simulink library "Driveline_ConnectFRDiffFDiffR"  (R2019a)
settings: Solver=VariableStepAuto  StartTime=0.0  StopTime=10.0  RelTol=1e-3
undefined symbols (not defined in the file): Driveline
libraries: sm_car_lib x6, fl_lib x4, sdl_lib x2
Description:
  | Component of Simscape Vehicle Templates Library
  | 
  | Copyright 2018-2020 The MathWorks, Inc.
settings Model: Creator=smiller  LastModifiedBy=smiller
settings DataIOCC: ReturnWorkspaceOutputs=off
settings DebuggingCC: ArithmeticOperatorsInVariantConditions=warning

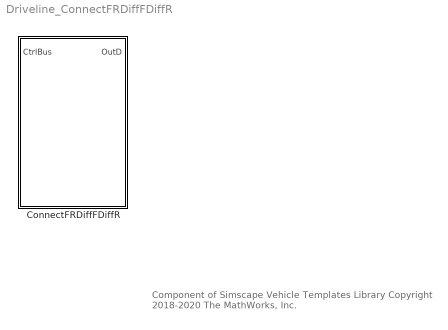
== system Driveline_ConnectFRDiffFDiffR ==
  note: Component of Simscape Vehicle Templates Library
      | Copyright 2018-2020 The MathWorks, Inc.
  ConnectFRDiffFDiffR : Subsystem  Tag=PublishSubsystem  VariantControl=ConnectFRDiffFDiffR  mask(Driveline, Connected Front and Rear){InitTriggerDropdown=0}
      mask prompts: InitTriggerDropdown "Initialization Trigger Dropdown"
      mask help: Models front and rear drivelines connected by a viscous coupling.
      mask init:
      | curblk = gcb;
      | 
      | % Trigger Mask Initialization for 
      | % variant subsystems below this level
      | sm_car_lib_maskInitTrigger(curblk);
      mask TypeOptions InitTriggerDropdown: 0 | 1
      mask Display: image('sm_car_vehicle_driveline_connectfrdifffdiffr_IMAGE.png');

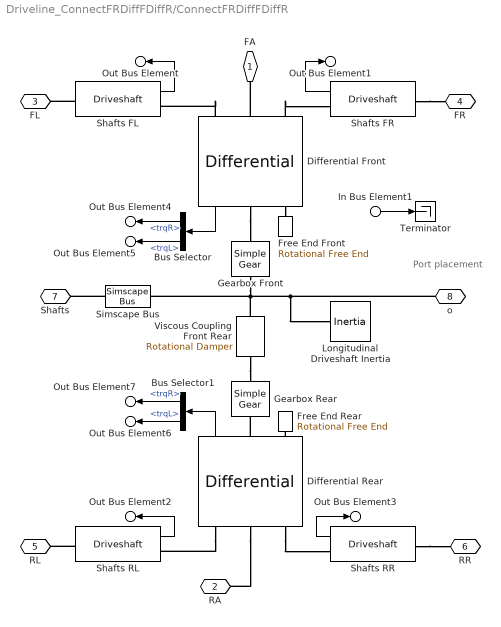
== system Driveline_ConnectFRDiffFDiffR/ConnectFRDiffFDiffR ==
  note: Port
      | placement
  In Bus Element1 : Inport  PortName=CtrlBus
  Bus Selector : BusSelector  OutputSignals=trqR,trqL
  Bus Selector1 : BusSelector  OutputSignals=trqR,trqL
  Differential Front : sm_car_lib/Driveline/Differential  VariantControl=Variant1  Differential=Driveline.DifferentialF  VariantLabel=Driveline.DifferentialF.class.Value  InitTriggerDropdown=0
      settings: AttributesFormatString=%<ActiveVariant>
  Differential Rear : sm_car_lib/Driveline/Differential  VariantControl=Variant1  Differential=Driveline.DifferentialR  VariantLabel=Driveline.DifferentialR.class.Value  InitTriggerDropdown=0
      settings: AttributesFormatString=%<ActiveVariant>
  Free End Front : fl_lib/Mechanical/Rotational Elements/Rotational Free End  w_specify=off  w_priority=None  w=0 rad/s  w_nominal_specify=off  w_nominal_unit=rad/s  w_nominal_value=1
      settings: SourceProductName=Simscape  SourceProductBaseCode=SS
  Free End Rear : fl_lib/Mechanical/Rotational Elements/Rotational Free End  w_specify=off  w_priority=None  w=0 rad/s  w_nominal_specify=off  w_nominal_unit=rad/s  w_nominal_value=1
      settings: SourceProductName=Simscape  SourceProductBaseCode=SS
  Gearbox Front : sdl_lib/Gears/Simple Gear  ratio=Driveline.GearboxF.ratio.Value  rotation_direction=1  friction_model=1  T_noload=0.1 N*m  T_nom=5 N*m  efficiency_nom=0.8  efficiency=0.8  mu_visc=[0, 0] N*m/(rad/s)  w_thr=0.01 rad/s  pwr_thr=0.001 W  enable_faults=0  efficiency_fault=0.05  external_fault=simscape.enum.onoff.off  temporal_fault=0  fault_time=5 s  fault_angles=pi / 12 rad  report_fault=1  temperature_TLU=[280, 300, 320] K  load_TLU=[1, 5, 10] N*m  efficiency_TLU=[.95, .9, .85]  efficiency_TLU2=[.85, .8, .75; .95, .9, .85; .85, .8, .7]  thermal_mass=50 J/K  T_init=300 K
      settings: SourceProductName=Simscape Driveline
  Gearbox Rear : sdl_lib/Gears/Simple Gear  ratio=Driveline.GearboxR.ratio.Value  rotation_direction=1  friction_model=1  T_noload=0.1 N*m  T_nom=5 N*m  efficiency_nom=0.8  efficiency=0.8  mu_visc=[0, 0] N*m/(rad/s)  w_thr=0.01 rad/s  pwr_thr=0.001 W  enable_faults=0  efficiency_fault=0.05  external_fault=simscape.enum.onoff.off  temporal_fault=0  fault_time=5 s  fault_angles=pi / 12 rad  report_fault=1  temperature_TLU=[280, 300, 320] K  load_TLU=[1, 5, 10] N*m  efficiency_TLU=[.95, .9, .85]  efficiency_TLU2=[.85, .8, .75; .95, .9, .85; .85, .8, .7]  thermal_mass=50 J/K  T_init=300 K
      settings: SourceProductName=Simscape Driveline
  Longitudinal Driveshaft Inertia : fl_lib/Mechanical/Rotational Elements/Inertia  inertia=Driveline.DriveshaftLong.J.Value kg*m^2  w_specify=on  w_priority=None  w=0 rad/s  w_nominal_specify=off  w_nominal_unit=rad/s  w_nominal_value=1  t_specify=off  t_priority=None  t=0 N*m  t_nominal_specify=off  t_nominal_unit=N*m  t_nominal_value=1
  Shafts FL : sm_car_lib/Driveline/Driveshaft  VariantControl=Variant1  popup_leftRight=Left  Driveshaft=Driveline.DriveshaftFL  VariantLabel=Driveline.DriveshaftFL.class.Value  InitTriggerDropdown=0
      settings: AttributesFormatString=%<ActiveVariant>
  Shafts FR : sm_car_lib/Driveline/Driveshaft  VariantControl=Variant1  popup_leftRight=Right  Driveshaft=Driveline.DriveshaftFR  VariantLabel=Driveline.DriveshaftFR.class.Value  InitTriggerDropdown=0
      settings: AttributesFormatString=%<ActiveVariant>
  Shafts RL : sm_car_lib/Driveline/Driveshaft  VariantControl=Variant1  popup_leftRight=Left  Driveshaft=Driveline.DriveshaftRL  VariantLabel=Driveline.DriveshaftRL.class.Value  InitTriggerDropdown=0
      settings: AttributesFormatString=%<ActiveVariant>
  Shafts RR : sm_car_lib/Driveline/Driveshaft  VariantControl=Variant1  popup_leftRight=Right  Driveshaft=Driveline.DriveshaftRR  VariantLabel=Driveline.DriveshaftRR.class.Value  InitTriggerDropdown=0
      settings: AttributesFormatString=%<ActiveVariant>
  Simscape Bus : SimscapeBus  HierarchyStrings=ShaftF
  Terminator : Terminator
  Viscous Coupling Front Rear : fl_lib/Mechanical/Rotational Elements/Rotational Damper  D=Driveline.CouplingFR.d.Value N*m/(rad/s)  w_specify=off  w_priority=None  w=0 rad/s  w_nominal_specify=off  w_nominal_unit=rad/s  w_nominal_value=1  t_specify=off  t_priority=None  t=0 N*m  t_nominal_specify=off  t_nominal_unit=N*m  t_nominal_value=1
  FA : PMIOPort  Side=Left
  RA : PMIOPort  Port=2  Side=Right
  FL : PMIOPort  Port=3  Side=Left
  FR : PMIOPort  Port=4  Side=Right
  RL : PMIOPort  Port=5  Side=Left
  RR : PMIOPort  Port=6  Side=Right
  Shafts : PMIOPort  Port=7  Side=Left
  o : PMIOPort  Port=8  Side=Right
  Out Bus Element6 : Outport  PortName=OutD  Element=MDriveshaftRL
  Out Bus Element7 : Outport  PortName=OutD  Element=MDriveshaftRR
  Out Bus Element4 : Outport  PortName=OutD  Element=MDriveshaftFL
  Out Bus Element5 : Outport  PortName=OutD  Element=MDriveshaftFR
  Out Bus Element : Outport  PortName=OutD  Element=anDriveshaftFL
  Out Bus Element1 : Outport  PortName=OutD  Element=anDriveshaftFR
  Out Bus Element2 : Outport  PortName=OutD  Element=anDriveshaftRL
  Out Bus Element3 : Outport  PortName=OutD  Element=anDriveshaftRR
  wires:
  Shafts RL/1 -> Out Bus Element2/1
  Shafts FR/1 -> Out Bus Element1/1
  Shafts RR/1 -> Out Bus Element3/1
  Shafts FL/1 -> Out Bus Element/1
  Differential Front/1 -> Bus Selector/1
  Bus Selector1/1 -> Out Bus Element7/1  "<trqR>"
  Bus Selector1/2 -> Out Bus Element6/1  "<trqL>"
  Differential Rear/1 -> Bus Selector1/1
  Bus Selector/1 -> Out Bus Element4/1  "<trqR>"
  Bus Selector/2 -> Out Bus Element5/1  "<trqL>"
  In Bus Element1/1 -> Terminator/1
  connections:
  Viscous Coupling Front Rear/LConn1 -- Gearbox Rear/LConn1
  Gearbox Front/LConn1 -- Simscape Bus/LConn1 -- Viscous Coupling Front Rear/RConn1 -- Longitudinal Driveshaft Inertia/LConn1 -- o/RConn1
  Differential Rear/RConn2 -- Free End Rear/LConn1
  Differential Front/RConn2 -- Free End Front/LConn1
  Differential Front/LConn1 -- Shafts FL/RConn1
  Differential Front/LConn3 -- Shafts FR/RConn1
  Shafts FR/LConn1 -- FR/RConn1
  Shafts FL/LConn1 -- FL/RConn1
  Differential Front/LConn2 -- FA/RConn1
  Differential Rear/LConn2 -- RA/RConn1
  Differential Front/RConn1 -- Gearbox Front/RConn1
  Shafts RR/LConn1 -- RR/RConn1
  Shafts RL/LConn1 -- RL/RConn1
  Differential Rear/LConn3 -- Shafts RR/RConn1
  Differential Rear/LConn1 -- Shafts RL/RConn1
  Differential Rear/RConn1 -- Gearbox Rear/RConn1
  Simscape Bus/RConn1 -- Shafts/RConn1
